simulink model "Observateur_step2_bruits"  (R2019a)
settings: Solver=VariableStepAuto  StartTime=0.0  StopTime=2  RelTol=1e-3
undefined symbols (not defined in the file): A, Ao, B, Bo, C, Co, Ko, u0, uf, x0, xo0
libraries: simulink x1
settings Model: Creator=Alex  LastModifiedBy=Alex

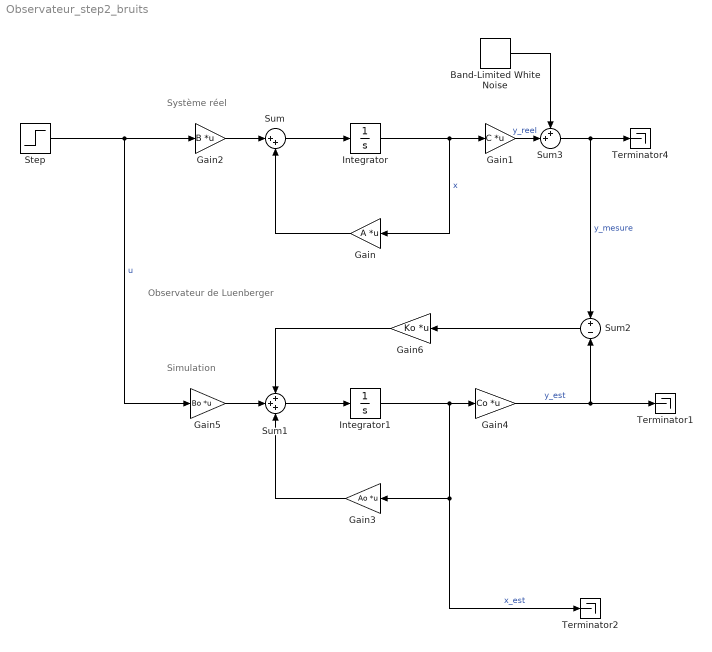
== system Observateur_step2_bruits ==
  note: Observateur de Luenberger
  note: Système réel
  note: Simulation
  "Band-Limited White Noise " : simulink/Sources/Band-Limited White Noise  Cov=[0.001]  Ts=0.001  seed=[23341]
  Gain : Gain  Gain=A  Multiplication=Matrix(K*u)
  Gain1 : Gain  Gain=C  Multiplication=Matrix(K*u)
  Gain2 : Gain  Gain=B  Multiplication=Matrix(K*u)
  Gain3 : Gain  Gain=Ao  Multiplication=Matrix(K*u)
  Gain4 : Gain  Gain=Co  Multiplication=Matrix(K*u)
  Gain5 : Gain  Gain=Bo  Multiplication=Matrix(K*u)
  Gain6 : Gain  Gain=Ko  Multiplication=Matrix(K*u)
  Integrator : Integrator  InitialCondition=x0
      settings: AttributesFormatString=Conditions intiales %<InitialCondition>
  Integrator1 : Integrator  InitialCondition=xo0
      settings: AttributesFormatString=Conditions intiales %<InitialCondition>
  Step : Step  Before=u0  After=uf  SampleTime=0
  Sum : Sum  Inputs=|++
  Sum1 : Sum  Inputs=+++
  Sum2 : Sum  Inputs=+-
  Sum3 : Sum  Inputs=++|
  Terminator1 : Terminator
  Terminator2 : Terminator
  Terminator4 : Terminator
  wires:
  Sum/1 -> Integrator/1
  Gain/1 -> Sum/2
  Integrator/1 -> Gain1/1, Gain/1  "x"
  Sum3/1 -> Terminator4/1, Sum2/1  "y_mesure"
  Gain2/1 -> Sum/1
  Step/1 -> Gain5/1, Gain2/1  "u"
  Integrator1/1 -> Terminator2/1, Gain3/1, Gain4/1  "x_est"
  Sum1/1 -> Integrator1/1
  Gain4/1 -> Terminator1/1, Sum2/2  "y_est"
  Sum2/1 -> Gain6/1
  Gain5/1 -> Sum1/2
  Gain3/1 -> Sum1/3
  Gain6/1 -> Sum1/1
  Gain1/1 -> Sum3/2  "y_reel"
  "Band-Limited White Noise "/1 -> Sum3/1
